simulink model "sqauare"  (Simulink 8.3)
settings: Solver=ode45  StartTime=0.0  StopTime=0.5  RelTol=1e-3
libraries: powerlib x8, powerlib_extras x1
settings Model: Creator=Singhal  LastModifiedBy=Singhal
settings DataIOCC: InspectSignalLogs=on
settings OptimizationCC: ExpressionDepthLimit=2147483647
settings DebuggingCC: FcnCallInpInsideContextMsg=UseLocalSettings

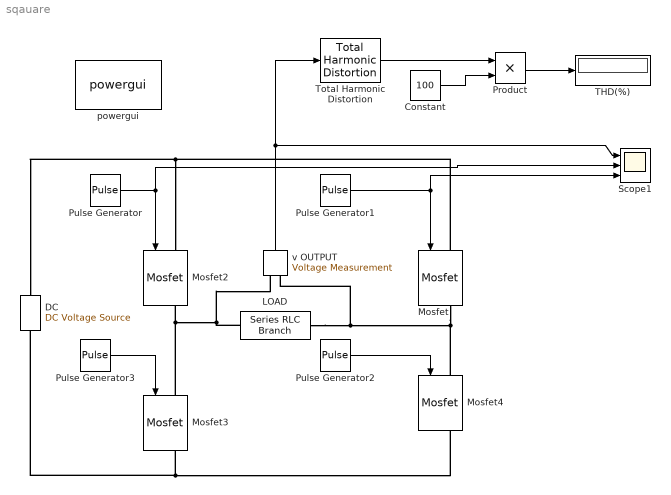
== system sqauare ==
  Constant : Constant  Value=100
  DC : powerlib/Electrical Sources/DC Voltage Source  Amplitude=100  Measurements=None
  LOAD : powerlib/Elements/Series RLC Branch  LConnTagsString=__new0  RConnTagsString=__new0  BranchType=R  Resistance=20  Inductance=1e-3  SetiL0=off  InitialCurrent=0  Capacitance=1e-6  Setx0=off  InitialVoltage=0  Measurements=None
  Mosfet{,2..4} (4 alike) : powerlib/Power Electronics/Mosfet  Ron=0.1  Lon=0  Rd=0.01  Vfd=0  IC=0  Rs=1e5  Cs=inf  Measurements=on
  Product : Product  RndMeth=Zero
  Pulse Generator : DiscretePulseGenerator  PulseType=Time based  Period=0.02  PulseWidth=50
  Pulse Generator1 : DiscretePulseGenerator  PulseType=Time based  Period=0.02  PulseWidth=50  PhaseDelay=0.01
  Pulse Generator2 : DiscretePulseGenerator  PulseType=Time based  Period=0.02  PulseWidth=50
  Pulse Generator3 : DiscretePulseGenerator  PulseType=Time based  Period=0.02  PulseWidth=50  PhaseDelay=0.01
  Scope1 : Scope  NumInputPorts=3
      settings: YMin=-100~-5~-5  YMax=100~5~5
  THD(%) : Display
  Total Harmonic Distortion : powerlib_extras/Measurements/Total Harmonic Distortion  f1=50
  powergui : powerlib/powergui  Priority=1  SimulationMode=Discrete  SolverType=Tustin  SampleTime=50e-6  frequency=60  SPID=off  DisableSnubberDevices=off  DisableRonSwitches=off  DisableVfSwitches=off  SwTol=0  Interpol=off  DisplayEquations=off  Ts=0  methode=off  frequencyindice=0  Pbase=100e6  ErrMax=1e-4  Iterations=50  UnitsV=kV  UnitsW=MW  FunctionMessages=off  echomessages=off  HookPort=off  EnableUseOfTLC=off  x0status=blocks  RestoreLinks=warning  ResistiveCurrentMeasurement=off  Frange=[0:2:500]  Ylog=off  Xlog=on  ShowGrid=off  save=off  variable=ZData  structure=ScopeData  ZoomFFT=on  StartTime=0.0  cycles=1  DisplayStyle=2  fundamental=50  FreqAxis=off  MaxFrequency=1000  frequencyindicesteady=1  RmsSteady=1  display=off
  v OUTPUT : powerlib/Measurements/Voltage Measurement  PhasorSimulation=off  OutputType=Complex  PSBequivalent=0
  wires:
  Constant/1 -> Product/2
  Total Harmonic Distortion/1 -> Product/1
  Product/1 -> THD(%)/1
  Pulse Generator/1 -> Mosfet2/1, Scope1/2
  Pulse Generator1/1 -> Mosfet/1, Scope1/3
  Pulse Generator2/1 -> Mosfet4/1
  Pulse Generator3/1 -> Mosfet3/1
  v OUTPUT/1 -> Scope1/1, Total Harmonic Distortion/1
  connections:
  Mosfet3/LConn1 -- Mosfet2/RConn1 -- LOAD/RConn1 -- v OUTPUT/LConn1
  Mosfet/LConn1 -- DC/RConn1 -- Mosfet2/LConn1
  DC/LConn1 -- Mosfet3/RConn1 -- Mosfet4/RConn1
  LOAD/LConn1 -- Mosfet4/LConn1 -- Mosfet/RConn1 -- v OUTPUT/LConn2
